simulink model "UAV"  (R2024a)
settings: Solver=FixedStepAuto  StartTime=0  StopTime=inf  MaxStep=0.01  RelTol=1e-4
values from neighbouring files (symbols this model uses):
  actuatorCentres = 0.0    [data.sldd]
  datcom1 : value not decoded    [data.sldd]
  deflectionLimits = -10.0    [data.sldd]
  loggingSampleTime = 1.0    [data.sldd]
  sensorSampleTime = 0.02    [data.sldd]
  vehicle = 1.23    [data.sldd]
undefined symbols (not defined in the file or in its folder): aeroCoeff, aMode, DiscIntNeverNeededParam, Discrete, Earth, HDBK, MIL, Newton, pa28, Raphson, Time, WGS84
libraries: slpidlib x20, simulink_extras x15, simulink x13, arduinolib x8, aerolibasang x5, aerolibactuator x4, aerolibutil x4, aerolibtransform2 x4, sharedtransform x3, ctrlSharedLib x3, aerolibadyn x3, dspstat3 x2
(part 1 of 5)
settings Model: DataDictionary=data.sldd  EnableAccessToBaseWorkspace=off  VariantConfigurationObject=Variants  SnapshotBufferSize=2  SnapshotInterval=1  PacingRate=10  ExtModeTrigDuration=2  Creator=Aliak  LastModifiedBy=abdul
settings SolverCC: AlgebraicLoopSolver=TrustRegion  SolverResetMethod=Robust  MinimalZcImpactIntegration=on
settings OptimizationCC: DefaultParameterBehavior=Inlined  UseDivisionForNetSlopeComputation=on  GainParamInheritBuiltInType=on  UseFloatMulNetSlope=on  DefaultUnderspecifiedDataType=single  UseSpecifiedMinMax=on  InlineInvariantSignals=on  EnhancedBackFolding=on  CachingGlobalReferences=on  ActiveStateOutputEnumStorageType=Smallest  ZeroExternalMemoryAtStartup=off  ZeroInternalMemoryAtStartup=off  EfficientFloat2IntCast=on  EfficientMapNaN2IntZero=off  LifeSpan=0.2  MaxStackSize=64  SimCompilerOptimization=on  OptimizeBlockOrder=speed  DifferentSizesBufferReuse=on  EfficientTunableParamExpr=on
settings DebuggingCC: ConsistencyChecking=warning  ReadBeforeWriteMsg=DisableAll  WriteAfterWriteMsg=DisableAll  WriteAfterReadMsg=DisableAll  SolverPrmCheckMsg=warning  ParameterTunabilityLossMsg=error  UnconnectedInputMsg=warning  UnconnectedOutputMsg=warning  UnconnectedLineMsg=warning  UniqueDataStoreMsg=error  BusObjectLabelMismatch=error  StateNameClashWarn=warning  ForceCombineOutputUpdateInSim=on  ArithmeticOperatorsInVariantConditions=warning
settings HardwareCC: ProdBitPerInt=16  ProdBitPerPointer=16  ProdBitPerSizeT=16  ProdBitPerPtrDiffT=16  ProdLargestAtomicFloat=None  ProdWordSize=8  ProdLongLongMode=on  ProdHWDeviceType=Atmel->AVR  TargetBitPerPointer=64  TargetBitPerSizeT=64  TargetBitPerPtrDiffT=64  TargetLongLongMode=on  TargetIntDivRoundTo=Zero  TargetEndianess=LittleEndian  TargetWordSize=64  TargetHWDeviceType=MATLAB Host
settings ModelReferenceCC: UpdateModelReferenceTargets=IfOutOfDate  EnableRefExpFcnMdlSchedulingChecks=on  EnableParallelModelReferenceBuilds=on  ModelReferenceMinAlgLoopOccurrences=on
settings SFSimCC: SFSimEcho=off  SimParseCustomCode=off  MATLABDynamicMemAlloc=off  CustomCodeUndefinedFunction=UseInterfaceOnly
settings RTWCC: Description=Embedded Coder  SystemTargetFile=ert.tlc  HardwareBoard=Arduino Uno  TemplateMakefile=ert_default_tmf  GenerateReport=on  Toolchain=Arduino AVR  BuildConfiguration=Faster Runs  IncludeHyperlinkInReport=on  LaunchReport=on  GenerateTraceInfo=on  GenerateTraceReport=on  GenerateTraceReportSl=on  GenerateTraceReportSf=on  GenerateTraceReportEml=on  GPUComputeCapability=3.5
settings CodeAppCC: ForceParamTrailComments=on  IgnoreCustomStorageClasses=off  OperatorAnnotations=on  SimulinkDataObjDesc=on  SFDataObjDesc=on  InsertBlockDesc=on
settings ERTTargetCC: TargetLangStandard=C99 (ISO)  CodeReplacementLibrary=GNU C99 extensions  UtilityFuncGeneration=Shared location  CombineSignalStateStructs=on  SuppressErrorStatus=on  SupportNonFinite=off  SupportContinuousTime=on  SupportVariableSizeSignals=on  InlinedParameterPlacement=NonHierarchical

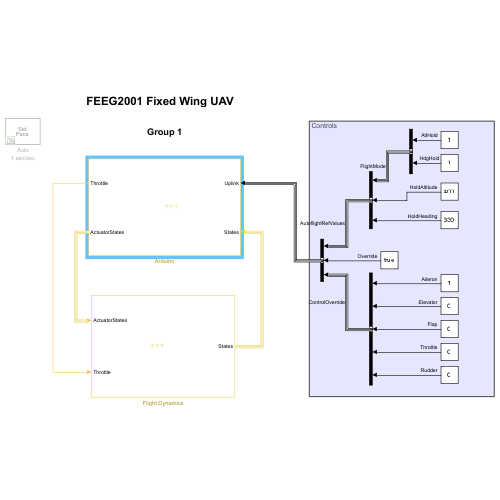
[thumbnail: Simulink's stored preview of the top-level diagram]
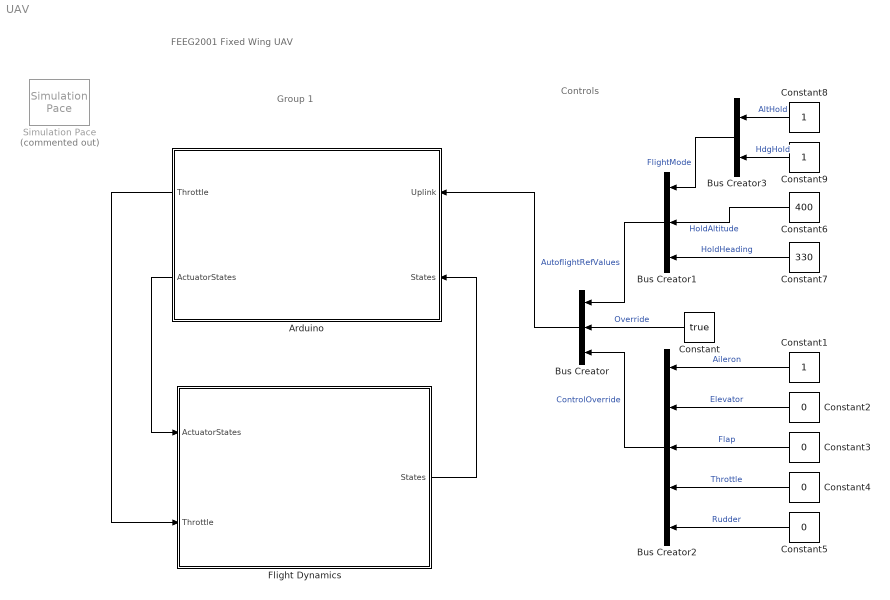
== system UAV ==
  note: Controls
  note: Group 1
  note: FEEG2001 Fixed Wing UAV
  Arduino : Subsystem
      mask Display: image('a000066_featured_1_.jpg');
  Bus Creator : BusCreator  Inputs=3  OutDataTypeStr=Bus: Uplink
  Bus Creator1 : BusCreator  Inputs=3  OutDataTypeStr=Bus: AutoflightDemandedValues
  Bus Creator2 : BusCreator  Inputs=5  OutDataTypeStr=Bus: ControlOverrides
  Bus Creator3 : BusCreator  Inputs=2
  Constant : Constant  Value=true  OutDataTypeStr=boolean
  Constant1 : Constant  OutDataTypeStr=single
  Constant{2..5} (4 alike) : Constant  Value=0  OutDataTypeStr=single
  Constant6 : Constant  Value=400  OutDataTypeStr=single
  Constant7 : Constant  Value=330  OutDataTypeStr=single
  Constant8 : Constant  OutDataTypeStr=single
  Constant9 : Constant  OutDataTypeStr=single
  Flight Dynamics : Subsystem
      mask Display: image('MQ-9-Reaper-armed-UAV.jpg');
  Simulation Pace : aerolibanimutils/Simulation Pace  Commented=on  SimulationPace=1  SleepMode=Auto  OutputPaceError=off  SampleTime=sensorSampleTime
  wires:
  Arduino/2(ActuatorStates) -> Flight Dynamics/1(ActuatorStates)
  Bus Creator/1 -> Arduino/1(Uplink)
  Flight Dynamics/1(States) -> Arduino/2(States)
  Arduino/1(Throttle) -> Flight Dynamics/2(Throttle)
  Bus Creator1/1 -> Bus Creator/1  "AutoflightRefValues"
  Constant/1 -> Bus Creator/2  "Override"
  Bus Creator2/1 -> Bus Creator/3  "ControlOverride"
  Constant1/1 -> Bus Creator2/1  "Aileron"
  Constant2/1 -> Bus Creator2/2  "Elevator"
  Constant3/1 -> Bus Creator2/3  "Flap"
  Constant4/1 -> Bus Creator2/4  "Throttle"
  Constant5/1 -> Bus Creator2/5  "Rudder"
  Bus Creator3/1 -> Bus Creator1/1  "FlightMode"
  Constant6/1 -> Bus Creator1/2  "HoldAltitude"
  Constant7/1 -> Bus Creator1/3  "HoldHeading"
  Constant8/1 -> Bus Creator3/1  "AltHold"
  Constant9/1 -> Bus Creator3/2  "HdgHold"

== system UAV/Arduino ==
  Uplink : Inport
  States : Inport  Port=2
  Actuators : Subsystem  Variant=on  VariantControlMode=label  LabelModeActiveChoice=SimType == 0
  Bus Selector : BusSelector  OutputSignals=Throttle
  Communications : Subsystem
  Flight Control : Subsystem  Variant=on  VariantControlMode=label  VariantControl=Variant1  LabelModeActiveChoice=SimType==0
  Rate Transition : RateTransition  OutPortSampleTime=loggingSampleTime
  Sensors : Subsystem  Variant=on  VariantControlMode=label  VariantControl=Variant1  LabelModeActiveChoice=SimType==0
  Telemetry and Errors : Subsystem  Variant=on  VariantControlMode=label  VariantControl=Variant1  LabelModeActiveChoice=SecArd == 0
  Throttle : Outport  VectorParamsAs1DForOutWhenUnconnected=off
  ActuatorStates : Outport  Port=2  VectorParamsAs1DForOutWhenUnconnected=off
  wires:
  Uplink/1 -> Communications/1(Uplink)
  States/1 -> Sensors/1(States)
  Communications/1(Demands) -> Flight Control/1("Demands ")
  Flight Control/1(" Commands") -> Bus Selector/1, Actuators/1(Commands)
  Rate Transition/1 -> Telemetry and Errors/1("Sensors ")
  Bus Selector/1 -> Throttle/1  "<Throttle>"
  Actuators/1(ActuatorStates) -> ActuatorStates/1
  Sensors/1(" Sensors") -> Flight Control/2("Sensors "), Rate Transition/1

== system UAV/Flight Dynamics ==
  ActuatorStates : Inport
  Throttle : Inport  Port=2
  6DOF EOM : Subsystem  VariantControl=eom3DOF
  Coeff Model : Subsystem  Commented=on  VariantControl=AeroModel==2
  DATCOM Model : Subsystem  TreatAsAtomicUnit=on  VariantControl=AeroModel==1
      settings: MinAlgLoopOccurrences=on
  Environment : Subsystem
  Propulsion : Subsystem
      settings: RTWSystemCode=Inline
  Sum1 : Sum  Inputs=|++  InputSameDT=on  SaturateOnIntegerOverflow=on  OutDataTypeStr=Inherit: Same as first input
  Sum2 : Sum  Inputs=|++  InputSameDT=on  SaturateOnIntegerOverflow=on  OutDataTypeStr=Inherit: Same as first input
  Visualization : Subsystem
  States : Outport  OutDataTypeStr=Bus: States  VectorParamsAs1DForOutWhenUnconnected=off
  wires:
  Sum2/1 -> 6DOF EOM/2(Forces)
  Propulsion/1(F) -> Sum2/2
  Propulsion/2(M) -> Sum1/2
  Sum1/1 -> 6DOF EOM/3(Moments)
  Throttle/1 -> Propulsion/1(cmd)
  ActuatorStates/1 -> DATCOM Model/3(ActuatorStates)
  DATCOM Model/1(F) -> Sum2/1
  DATCOM Model/2(M) -> Sum1/1
  Environment/1(Env) -> 6DOF EOM/1(Env), DATCOM Model/1(Env)
  6DOF EOM/1(DCMbe) -> Environment/2(DCMbe)
  6DOF EOM/2(States) -> Environment/1(States), Visualization/1(States), DATCOM Model/2(States), States/1

== system UAV/Arduino/Actuators ==
  Commands : Inport
  Model Actuators : Subsystem  VariantControl=SimType == 0
  Real Actuators : Subsystem  VariantControl=SimType == 1
  ActuatorStates : Outport  VectorParamsAs1DForOutWhenUnconnected=off

== system UAV/Arduino/Communications ==
  Uplink : Inport  OutDataTypeStr=Bus: Uplink
  Bus Creator : BusCreator  Inputs=5  OutDataTypeStr=Bus: Demands
      settings: InheritFromInputs=off
  Bus Selector : BusSelector  OutputSignals=AutoflightRefValues,Override,ControlOverride
  Bus Selector1 : BusSelector  OutputSignals=FlightMode,HoldAltitude,HoldHeading
  Demands : Outport  OutDataTypeStr=Bus: Demands  VectorParamsAs1DForOutWhenUnconnected=off
  wires:
  Uplink/1 -> Bus Selector/1
  Bus Selector/1 -> Bus Selector1/1  "<AutoflightRefValues>"
  Bus Selector1/1 -> Bus Creator/1  "<FlightMode>"
  Bus Selector1/2 -> Bus Creator/2  "<HoldAltitude>"
  Bus Selector1/3 -> Bus Creator/3  "<HoldHeading>"
  Bus Creator/1 -> Demands/1
  Bus Selector/3 -> Bus Creator/5  "<ControlOverride>"
  Bus Selector/2 -> Bus Creator/4  "<Override>"

== system UAV/Arduino/Flight Control ==
  "Demands " : Inport
  "Sensors " : Inport  Port=2
  Model Flight Control : Subsystem  VariantControl=SimType==0
  Real Flight Control : Subsystem  VariantControl=SimType==1
  " Commands" : Outport  VectorParamsAs1DForOutWhenUnconnected=off

== system UAV/Arduino/Sensors ==
  States : Inport
  Model Sensors : Subsystem  VariantControl=SimType==0
  Real Sensors : Subsystem  VariantControl=SimType==1
  " Sensors" : Outport  OutDataTypeStr=Bus: Sensors  VectorParamsAs1DForOutWhenUnconnected=off

== system UAV/Arduino/Telemetry and Errors ==
  "Sensors " : Inport  OutDataTypeStr=Bus: Sensors  SampleTime=loggingSampleTime
  SD_Logging : Subsystem  VariantControl=SecArd == 1
  Simulink Logging : Subsystem  VariantControl=SecArd == 0

== system UAV/Flight Dynamics/6DOF EOM ==
  Bus Element In : Inport  PortName=Env  Element=g
  Forces : Inport  Port=2
  Moments : Inport  Port=3
  6DOF (Euler Angles) : shared6dof/6DOF (Euler Angles)  units=Metric (MKS)  mtype=Fixed  rep=Quaternion  xme_0=initConditions.x0  Vm_0=initConditions.v0  eul_0=initConditions.euler0  pm_0=initConditions.w0  mass_0=vehicle.mass  mass_e=0.5  mass_f=2.0  inertia=vehicle.inertia  inertia_e=eye(3)  inertia_f=2*eye(3)  k_quat=1.0  vre_flag=on  abi_flag=on  aMode=0  xme_statename=''  Vm_statename=''  eul_statename=''  quat_statename=''  pm_statename=''  mass_statename=''
  Cast To Double : DataTypeConversion  OutDataTypeStr=double  SaturateOnIntegerOverflow=off  RndMeth=Floor
  Gain : Gain  Gain=vehicle.mass
  Product : Product  Multiplication=Matrix(*)
  Sum2 : Sum  Inputs=++|  InputSameDT=on  SaturateOnIntegerOverflow=on  OutDataTypeStr=Inherit: Same as first input
  Terminator1 : Terminator
  DCMbe : Outport  VectorParamsAs1DForOutWhenUnconnected=off
  Bus Element Out : Outport  Port=2  VectorParamsAs1DForOutWhenUnconnected=off  PortName=States  Element=phi_theta_psi
  Bus Element Out1 : Outport  Port=2  VectorParamsAs1DForOutWhenUnconnected=off  PortName=States  Element=pqr
  Bus Element Out2 : Outport  Port=2  VectorParamsAs1DForOutWhenUnconnected=off  PortName=States  Element=omega_dot
  Bus Element Out15 : Outport  Port=2  VectorParamsAs1DForOutWhenUnconnected=off  PortName=States  Element=X_e
  Bus Element Out16 : Outport  Port=2  VectorParamsAs1DForOutWhenUnconnected=off  PortName=States  Element=V_b
  Bus Element Out17 : Outport  Port=2  VectorParamsAs1DForOutWhenUnconnected=off  PortName=States  Element=A_be
  Bus Element Out3 : Outport  Port=2  VectorParamsAs1DForOutWhenUnconnected=off  PortName=States  Element=V_e
  wires:
  6DOF (Euler Angles)/4 -> DCMbe/1, Product/1
  6DOF (Euler Angles)/1 -> Cast To Double/1
  Bus Element In/1 -> Gain/1
  6DOF (Euler Angles)/9 -> Bus Element Out17/1
  6DOF (Euler Angles)/7 -> Bus Element Out2/1
  6DOF (Euler Angles)/6 -> Bus Element Out1/1
  6DOF (Euler Angles)/5 -> Bus Element Out16/1
  6DOF (Euler Angles)/3 -> Bus Element Out/1
  6DOF (Euler Angles)/2 -> Bus Element Out15/1
  Gain/1 -> Product/2
  Sum2/1 -> 6DOF (Euler Angles)/1
  Product/1 -> Sum2/1
  6DOF (Euler Angles)/8 -> Terminator1/1
  Moments/1 -> 6DOF (Euler Angles)/2
  Forces/1 -> Sum2/2
  Cast To Double/1 -> Bus Element Out3/1

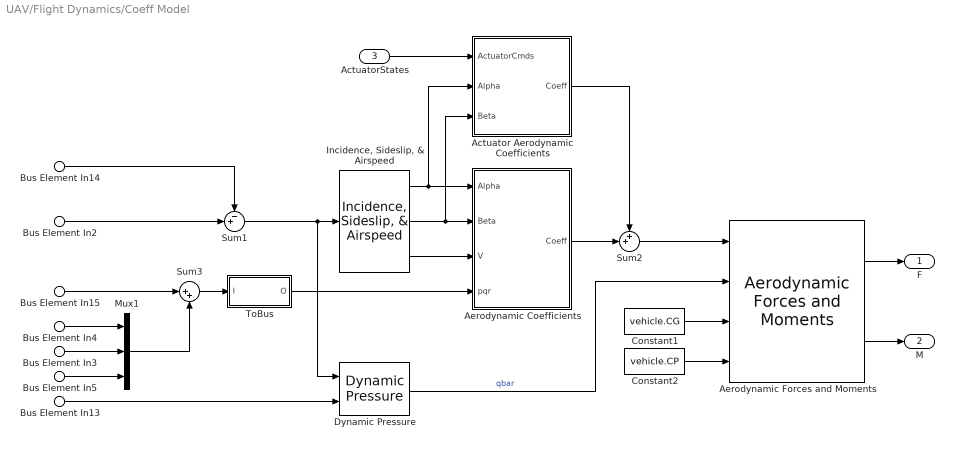
== system UAV/Flight Dynamics/Coeff Model ==
  Bus Element In13 : Inport  PortName=Env  Element=AirDensity
  Bus Element In14 : Inport  PortName=Env  Element=WindVelocity
  Bus Element In15 : Inport  PortName=Env  Element=WindAngularRates
  Bus Element In3 : Inport  Port=2  PortName=States  Element=q
  Bus Element In4 : Inport  Port=2  PortName=States  Element=p
  Bus Element In5 : Inport  Port=2  PortName=States  Element=r
  Bus Element In2 : Inport  Port=2  PortName=States  Element=V_e
  ActuatorStates : Inport  Port=3  OutDataTypeStr=Bus: ActuatorStates
  Actuator Aerodynamic Coefficients : Subsystem
  Aerodynamic Coefficients : Subsystem
  Aerodynamic Forces and Moments : aerolibadyn/Aerodynamic Forces and Moments   inputAxes=Body  outputForceAxes=Body  outputMomentAxes=Body  S=vehicle.wingarea  b=vehicle.wingspan  cbar=vehicle.aclength
  Constant1 : Constant  Value=vehicle.CG
  Constant2 : Constant  Value=vehicle.CP
  Dynamic Pressure : aerolibasang/Dynamic Pressure
  "Incidence, Sideslip, & Airspeed" : aerolibasang/Incidence, Sideslip, & Airspeed
  Mux1 : Mux  Inputs=3
  Sum1 : Sum  Inputs=-+|  InputSameDT=on  SaturateOnIntegerOverflow=on  OutDataTypeStr=Inherit: Same as first input
  Sum2 : Sum  Inputs=++|
  Sum3 : Sum  Inputs=|++  InputSameDT=on  SaturateOnIntegerOverflow=on  OutDataTypeStr=Inherit: Same as first input
  ToBus : Subsystem
  F : Outport  Unit=N  VectorParamsAs1DForOutWhenUnconnected=off
  M : Outport  Port=2  Unit=N*m  VectorParamsAs1DForOutWhenUnconnected=off
  wires:
  ActuatorStates/1 -> Actuator Aerodynamic Coefficients/1(ActuatorCmds)
  Bus Element In14/1 -> Sum1/1
  Bus Element In2/1 -> Sum1/2
  Mux1/1 -> Sum3/2
  Bus Element In15/1 -> Sum3/1
  Bus Element In5/1 -> Mux1/3
  Bus Element In3/1 -> Mux1/2
  Bus Element In4/1 -> Mux1/1
  Actuator Aerodynamic Coefficients/1(Coeff) -> Sum2/1
  Aerodynamic Coefficients/1(Coeff) -> Sum2/2
  ToBus/1(O) -> Aerodynamic Coefficients/4(pqr)
  Sum1/1 -> Dynamic Pressure/1, "Incidence, Sideslip, & Airspeed"/1
  Dynamic Pressure/1 -> Aerodynamic Forces and Moments/2  "qbar"
  Sum3/1 -> ToBus/1(I)
  Bus Element In13/1 -> Dynamic Pressure/2
  "Incidence, Sideslip, & Airspeed"/3 -> Aerodynamic Coefficients/3(V)
  "Incidence, Sideslip, & Airspeed"/2 -> Aerodynamic Coefficients/2(Beta), Actuator Aerodynamic Coefficients/3(Beta)
  Aerodynamic Forces and Moments/2 -> M/1
  Aerodynamic Forces and Moments/1 -> F/1
  Constant2/1 -> Aerodynamic Forces and Moments/4
  Constant1/1 -> Aerodynamic Forces and Moments/3
  Sum2/1 -> Aerodynamic Forces and Moments/1
  "Incidence, Sideslip, & Airspeed"/1 -> Actuator Aerodynamic Coefficients/2(Alpha), Aerodynamic Coefficients/1(Alpha)

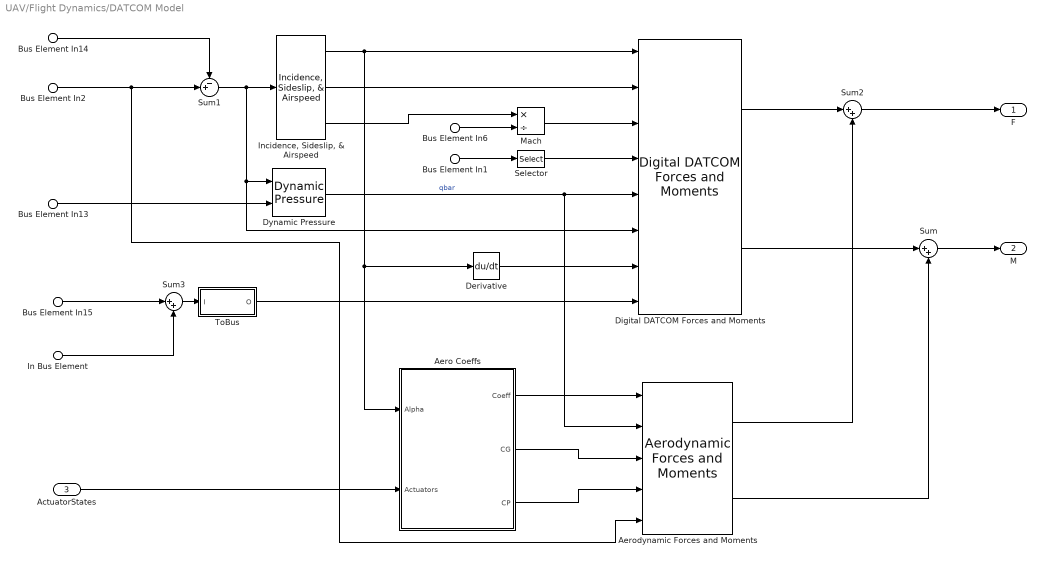
== system UAV/Flight Dynamics/DATCOM Model ==
  Bus Element In13 : Inport  PortName=Env  Element=AirDensity
  Bus Element In14 : Inport  PortName=Env  Element=WindVelocity
  Bus Element In15 : Inport  PortName=Env  Element=WindAngularRates
  Bus Element In6 : Inport  PortName=Env  Element=a
  Bus Element In2 : Inport  Port=2  PortName=States  Element=V_e
  Bus Element In1 : Inport  Port=2  PortName=States  Element=X_e
  In Bus Element : Inport  Port=2  PortName=States  Element=pqr
  ActuatorStates : Inport  Port=3  OutDataTypeStr=Bus: ActuatorStates
  Aero Coeffs : Subsystem
  "Aerodynamic Forces and Moments " : aerolibadyn/Aerodynamic Forces and Moments   inputAxes=Wind  outputForceAxes=Body  outputMomentAxes=Body  S=vehicle.wingarea  b=vehicle.wingspan  cbar=vehicle.cbar
  Derivative : Derivative  CoefficientInTFapproximation=1
  Digital DATCOM Forces and Moments : aerolibadyn/Digital DATCOM Forces and Moments  units=Metric (MKS)  dcase=datcom1{3}  fmode=Body  buildno=0  imethod=Linear  emethod=Linear  rmethod=Linear Extrapolation  action=Warning
  Dynamic Pressure : aerolibasang/Dynamic Pressure
  "Incidence, Sideslip, & Airspeed" : aerolibasang/Incidence, Sideslip, & Airspeed
  Mach : Product  Inputs=*/
  Selector : Selector  IndexMode=Zero-based  InputPortWidth=3  IndexOptions=Index vector (dialog)  Indices=[2]  OutputSizes=1
  Sum : Sum  Inputs=|++
  Sum1 : Sum  Inputs=-+|  InputSameDT=on  SaturateOnIntegerOverflow=on  OutDataTypeStr=Inherit: Same as first input
  Sum2 : Sum  Inputs=|++
  Sum3 : Sum  Inputs=|++  InputSameDT=on  SaturateOnIntegerOverflow=on  OutDataTypeStr=Inherit: Same as first input
  ToBus : Subsystem
  F : Outport  Unit=N  VectorParamsAs1DForOutWhenUnconnected=off
  M : Outport  Port=2  Unit=N*m  VectorParamsAs1DForOutWhenUnconnected=off
  wires:
  Bus Element In14/1 -> Sum1/1
  Bus Element In2/1 -> "Aerodynamic Forces and Moments "/5, Sum1/2
  In Bus Element/1 -> Sum3/2
  Bus Element In15/1 -> Sum3/1
  Sum1/1 -> "Incidence, Sideslip, & Airspeed"/1, Digital DATCOM Forces and Moments/6, Dynamic Pressure/1
  Sum3/1 -> ToBus/1(I)
  Bus Element In13/1 -> Dynamic Pressure/2
  "Incidence, Sideslip, & Airspeed"/3 -> Mach/1
  Digital DATCOM Forces and Moments/2 -> Sum/1
  Digital DATCOM Forces and Moments/1 -> Sum2/1
  Dynamic Pressure/1 -> "Aerodynamic Forces and Moments "/2, Digital DATCOM Forces and Moments/5  "qbar"
  Bus Element In1/1 -> Selector/1
  Selector/1 -> Digital DATCOM Forces and Moments/4
  Bus Element In6/1 -> Mach/2
  ActuatorStates/1 -> Aero Coeffs/2(Actuators)
  "Incidence, Sideslip, & Airspeed"/2 -> Digital DATCOM Forces and Moments/2
  "Incidence, Sideslip, & Airspeed"/1 -> Digital DATCOM Forces and Moments/1, Derivative/1, Aero Coeffs/1(Alpha)
  Aero Coeffs/1(Coeff) -> "Aerodynamic Forces and Moments "/1
  Aero Coeffs/2(CG) -> "Aerodynamic Forces and Moments "/3
  Aero Coeffs/3(CP) -> "Aerodynamic Forces and Moments "/4
  Sum/1 -> M/1
  "Aerodynamic Forces and Moments "/2 -> Sum/2
  Sum2/1 -> F/1
  "Aerodynamic Forces and Moments "/1 -> Sum2/2
  ToBus/1(O) -> Digital DATCOM Forces and Moments/8
  Derivative/1 -> Digital DATCOM Forces and Moments/7
  Mach/1 -> Digital DATCOM Forces and Moments/3

== system UAV/Flight Dynamics/Environment ==
  States : Inport
  DCMbe : Inport  Port=2
  Bus Creator : BusCreator  Inputs=5
  Bus Selector : BusSelector  OutputSignals=X_e,V_e
  Dryden Wind Turbulence Model (Discrete (-q +r)) : aerolibwind2/Dryden Wind Turbulence Model  (Continuous (+q -r))  units=Metric (MKS)  spec=MIL-HDBK-1797  model=Discrete Dryden (-q +r)  W20=1  Wdeg=250  TurbProb=10^-1  L_high=533.4  Wingspan=1.8  ts=sensorSampleTime  Seed=[23341 23342 23343 23344]  T_on=off
  Lapse Rate Model : aerolibatmos2/ISA Atmosphere Model  useExtended=off  action=Warning  custom=off  viscosityOut=off  g=9.80665  gamma=1.4  R=287.0531  L=0.0065  h_trop=11000  h_strat=20000  rho0=1.225  P0=101325  T0=288.15  h0=0  S=110.4  Tref=273.15  muref=1.716e-5
  Selector : Selector  IndexMode=Zero-based  InputPortWidth=3  IndexOptions=Index vector (dialog)  Indices=[0]  OutputSizes=1
  Selector1 : Selector  IndexMode=Zero-based  InputPortWidth=3  IndexOptions=Index vector (dialog)  Indices=[0]  OutputSizes=1
  Terminator : Terminator
  Terminator1 : Terminator
  g : Constant  Value=[0 0 9.80665]
  Env : Outport  VectorParamsAs1DForOutWhenUnconnected=off
  wires:
  States/1 -> Bus Selector/1
  Bus Creator/1 -> Env/1
  Selector/1 -> Dryden Wind Turbulence Model (Discrete (-q +r))/1, Lapse Rate Model/1
  Bus Selector/1 -> Selector/1  "<X_e>"
  Lapse Rate Model/4 -> Bus Creator/2  "AirDensity"
  Lapse Rate Model/2 -> Bus Creator/1  "a"
  g/1 -> Bus Creator/3  "g"
  DCMbe/1 -> Dryden Wind Turbulence Model (Discrete (-q +r))/3
  Bus Selector/2 -> Selector1/1  "<V_e>"
  Selector1/1 -> Dryden Wind Turbulence Model (Discrete (-q +r))/2
  Dryden Wind Turbulence Model (Discrete (-q +r))/1 -> Bus Creator/4  "WindVelocity"
  Dryden Wind Turbulence Model (Discrete (-q +r))/2 -> Bus Creator/5  "WindAngularRates"
  Lapse Rate Model/1 -> Terminator/1
  Lapse Rate Model/3 -> Terminator1/1

== system UAV/Flight Dynamics/Propulsion ==
  cmd : Inport  OutDataTypeStr=single
  Cast To Double : DataTypeConversion  OutDataTypeStr=double  SaturateOnIntegerOverflow=off  RndMeth=Floor
  Mux : Mux  Inputs=[1 2]
  Product : Product
  ThrustX : Lookup_n-D  NumberOfTableDimensions=1  LookupTableObject=''  BreakpointsForDimension1=(1/6)*(3+([-3:3]))  IndexSearchMethod=Linear search  BeginIndexSearchUsingPreviousIndexResult=on  Table=vehicle.thrust*(1+tanh([-3:3]))  ExtrapMethod=Clip  InternalRulePriority=Speed  InputSameDT=off
  ThrustYZ : Constant  Value=[0 0]'  SampleTime=-1
  Thrust_M1 : Constant  Value=[0 -0.06 0]  VectorParams1D=off  SampleTime=-1
  Vector Concatenate : Concatenate
  F : Outport  Unit=N  VectorParamsAs1DForOutWhenUnconnected=off
  M : Outport  Port=2  Unit=N*m  VectorParamsAs1DForOutWhenUnconnected=off
  wires:
  Thrust_M1/1 -> Product/2
  ThrustX/1 -> Mux/1, Vector Concatenate/2
  ThrustYZ/1 -> Vector Concatenate/1, Mux/2
  Mux/1 -> F/1
  cmd/1 -> Cast To Double/1
  Product/1 -> M/1
  Vector Concatenate/1 -> Product/1
  Cast To Double/1 -> ThrustX/1

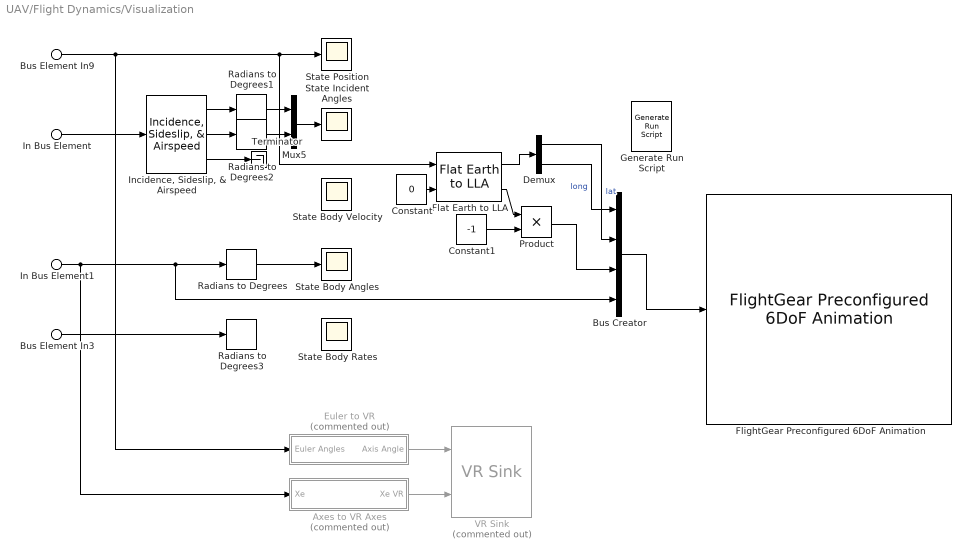
== system UAV/Flight Dynamics/Visualization ==
  Bus Element In3 : Inport  PortName=States  Element=pqr
  In Bus Element : Inport  PortName=States  Element=V_e
  In Bus Element1 : Inport  PortName=States  Element=phi_theta_psi
  Bus Element In9 : Inport  PortName=States  Element=X_e
  Axes to VR Axes : Subsystem  Commented=on
  Bus Creator : BusCreator  Inputs=4
  Constant : Constant  Value=0
  Constant1 : Constant  Value=-1
  Demux : Demux  Outputs=2
  Euler to VR : Subsystem  Commented=on
  Flat Earth to LLA : aerolibtransform2/Flat Earth to LLA  units=Metric (MKS)  ptype=Earth (WGS84)  F=1/298.257223563  R=6378137  refPosPort=off  LL0=[32.2476 15.1232]  psi=0
  FlightGear Preconfigured 6DoF Animation : aerolibfltsims/FlightGear Preconfigured 6DoF Animation  xFlightGearVersion=v2019.1  DestinationIpAddress=127.0.0.1  DestinationPort=5502  SampleTime=1/30  packetVersion=24
  Generate Run Script : aerolibfltsims/Generate Run Script  Architecture=Default  dataFlow=Send  GeometryModelName=pa28-161  AirportId=HL76  RunwayId=33  InitialAltitude=40  InitialHeading=330  OffsetDistance=0  OffsetAzimuth=0  InstallScenery=off  DisableShaders=off  OriginAddress=127.0.0.1  DestinationPort=5502  OriginPort=5505  LocalAddress=127.0.0.1  OutputFileName=runfg.bat  FlightGearBaseDirectory=E:\FlightGear 2020.3
  "Incidence, Sideslip, & Airspeed" : aerolibasang/Incidence, Sideslip, & Airspeed
  Mux5 : Mux  Inputs=2
  Product : Product
  Radians to Degrees{,1..3} (4 alike) : simulink_extras/Transformations/Radians to Degrees
  State Body Angles : Scope
  State Body Rates : Scope
  State Body Velocity : Scope
  State Incident Angles : Scope
  State Position : Scope
  Terminator : Terminator
  VR Sink : vrlib/VR Sink  Commented=on  InstantiateOnLoad=on  SampleTime=0.1  ViewEnable=on  RemoteChange=off  RemoteView=off  FieldsWritten=HL20.rotation.4.1.1.double#HL20.translation.3.1.1.double  WorldFileName=aeroblk_HL20.wrl  WorldDescription=aeroblk_HL20  AutoView=on  VideoDimensions=[]  AllowVariableSize=off  FigureProperties=[]
  wires:
  Mux5/1 -> State Incident Angles/1
  "Incidence, Sideslip, & Airspeed"/2 -> Radians to Degrees2/1
  "Incidence, Sideslip, & Airspeed"/1 -> Radians to Degrees1/1
  In Bus Element/1 -> "Incidence, Sideslip, & Airspeed"/1
  Bus Element In3/1 -> Radians to Degrees3/1
  "Incidence, Sideslip, & Airspeed"/3 -> Terminator/1
  Axes to VR Axes/1(Xe VR) -> VR Sink/2
  In Bus Element1/1 -> Bus Creator/4, Radians to Degrees/1, Axes to VR Axes/1(Xe)
  Euler to VR/1(Axis Angle) -> VR Sink/1
  Bus Element In9/1 -> Flat Earth to LLA/1, State Position/1, Euler to VR/1(Euler Angles)
  Radians to Degrees/1 -> State Body Angles/1
  Radians to Degrees1/1 -> Mux5/1
  Radians to Degrees2/1 -> Mux5/2
  Bus Creator/1 -> FlightGear Preconfigured 6DoF Animation/1
  Constant/1 -> Flat Earth to LLA/2
  Flat Earth to LLA/1 -> Demux/1
  Demux/1 -> Bus Creator/2  "lat"
  Demux/2 -> Bus Creator/1  "long"
  Constant1/1 -> Product/2
  Flat Earth to LLA/2 -> Product/1
  Product/1 -> Bus Creator/3

== system UAV/Arduino/Actuators/Model Actuators ==
  Commands : Inport
  Bus Creator : BusCreator  Inputs=4  OutDataTypeStr=Bus: ActuatorStates
  Bus Selector : BusSelector  OutputSignals=Aileron,Elevator,Rudder,Flap
  Cast To Double{,1..3} (4 alike) : DataTypeConversion  OutDataTypeStr=double  SaturateOnIntegerOverflow=off  RndMeth=Floor
  Constant : Constant  Value=0
  Linear Second-Order Actuator{,1..3} (4 alike) : aerolibactuator/Linear Second-Order Actuator  wn_fin=1  z_fin=0.05  fin_act_0=0  fin_act_vel=0
  Saturation : Saturate  UpperLimit=deflectionLimits.aileron.max  LowerLimit=deflectionLimits.aileron.min
  Saturation1 : Saturate  UpperLimit=deflectionLimits.elevator.max  LowerLimit=deflectionLimits.elevator.min
  Saturation2 : Saturate  UpperLimit=deflectionLimits.rudder.max  LowerLimit=deflectionLimits.rudder.min
  Saturation3 : Saturate  UpperLimit=deflectionLimits.flap.max  LowerLimit=deflectionLimits.flap.min
  Subtract{,1..3} (4 alike) : Sum  Inputs=+-
  ActuatorStates : Outport  VectorParamsAs1DForOutWhenUnconnected=off
  wires:
  Bus Selector/3 -> Subtract2/1  "<Rudder>"
  Bus Selector/4 -> Subtract3/1  "<Flap>"
  Bus Selector/1 -> Subtract1/1  "<Aileron>"
  Bus Selector/2 -> Subtract/1  "<Elevator>"
  Saturation1/1 -> Cast To Double1/1  "Elevator"
  Saturation/1 -> Cast To Double/1  "Aileron"
  Saturation2/1 -> Cast To Double2/1  "Rudder"
  Saturation3/1 -> Cast To Double3/1  "Flap"
  Bus Creator/1 -> ActuatorStates/1
  Commands/1 -> Bus Selector/1
  Subtract1/1 -> Saturation/1
  Subtract/1 -> Saturation1/1
  Subtract2/1 -> Saturation2/1
  Subtract3/1 -> Saturation3/1
  Constant/1 -> Subtract1/2, Subtract/2, Subtract2/2, Subtract3/2
  Cast To Double/1 -> Linear Second-Order Actuator/1
  Cast To Double1/1 -> Linear Second-Order Actuator1/1
  Cast To Double2/1 -> Linear Second-Order Actuator2/1
  Cast To Double3/1 -> Linear Second-Order Actuator3/1
  Linear Second-Order Actuator/1 -> Bus Creator/1  "Aileron"
  Linear Second-Order Actuator1/1 -> Bus Creator/2  "Elevator"
  Linear Second-Order Actuator2/1 -> Bus Creator/3  "Rudder"
  Linear Second-Order Actuator3/1 -> Bus Creator/4  "Flap"

== system UAV/Arduino/Actuators/Real Actuators ==
  Commands : Inport
  Aileron Servos : arduinolib/Standard Servo Write  pinNumber=servoPins.aileron.right  ServoIndex=0  blockPlatform=ARDUINO
  Bus Selector : BusSelector  OutputSignals=AileronCmd,ElevatorCmd,RudderCmd,FlapCmd
  Constant : Constant  Value=actuatorCentres.aileron.left
  Constant1 : Constant  Value=actuatorCentres.elevator.left
  Constant2 : Constant  Value=actuatorCentres.rudder
  Constant3 : Constant  Value=actuatorCentres.flap.left
  Elevator Servo : arduinolib/Standard Servo Write  pinNumber=servoPins.elevator.right  ServoIndex=0  blockPlatform=ARDUINO
  Flap Servo : arduinolib/Standard Servo Write  pinNumber=servoPins.flap.right  ServoIndex=0  blockPlatform=ARDUINO
  Initialize Function : Subsystem  TreatAsAtomicUnit=on
  Rudder Servo : arduinolib/Standard Servo Write  pinNumber=servoPins.rudder  ServoIndex=0  blockPlatform=ARDUINO
  Saturation : Saturate  Commented=through  UpperLimit=deflectionLimits.aileron.max  LowerLimit=deflectionLimits.aileron.min
  Saturation1 : Saturate  Commented=through  UpperLimit=deflectionLimits.elevator.max  LowerLimit=deflectionLimits.elevator.min
  Saturation2 : Saturate  Commented=through  UpperLimit=deflectionLimits.rudder.max  LowerLimit=deflectionLimits.rudder.min
  Saturation3 : Saturate  Commented=through  UpperLimit=deflectionLimits.flap.max  LowerLimit=deflectionLimits.flap.min
  Subtract{,1..3} (4 alike) : Sum  Inputs=-+
  wires:
  Saturation/1 -> Subtract/2
  Bus Selector/3 -> Saturation2/1  "<RudderCmd>"
  Commands/1 -> Bus Selector/1
  Bus Selector/4 -> Saturation3/1  "<FlapCmd>"
  Subtract3/1 -> Flap Servo/1
  Bus Selector/1 -> Saturation/1  "<AileronCmd>"
  Constant2/1 -> Subtract2/1
  Subtract2/1 -> Rudder Servo/1
  Saturation3/1 -> Subtract3/2
  Saturation2/1 -> Subtract2/2
  Saturation1/1 -> Subtract1/2
  Bus Selector/2 -> Saturation1/1  "<ElevatorCmd>"
  Subtract/1 -> Aileron Servos/1
  Subtract1/1 -> Elevator Servo/1
  Constant/1 -> Subtract/1
  Constant1/1 -> Subtract1/1
  Constant3/1 -> Subtract3/1

== system UAV/Arduino/Flight Control/Model Flight Control ==
  Demands : Inport  OutDataTypeStr=Bus: Demands
  Sensors : Inport  Port=2  OutDataTypeStr=Bus: Sensors
  Bus Creator : BusCreator  Inputs=5  OutDataTypeStr=Bus: Commands
      settings: InheritFromInputs=off
  Bus Selector : BusSelector  OutputSignals=ControlOverrides
  Bus Selector2 : BusSelector  OutputSignals=Aileron,Elevator,Flap,Throttle,Rudder
  Bus Selector3 : BusSelector  OutputSignals=Override
  Demux : Demux  Outputs=2
  Guidance States : Stateflow chart  Commented=on
  HDG_ALT : Subsystem
  NOT : Logic  Operator=NOT  IconShape=distinctive  AllPortsSameDT=off  OutDataTypeStr=boolean
  Saturation : Saturate  UpperLimit=deflectionLimits.aileron.max  LowerLimit=deflectionLimits.aileron.min
  Saturation1 : Saturate  UpperLimit=deflectionLimits.elevator.max  LowerLimit=deflectionLimits.elevator.min
  Stabilisation : Subsystem
  Sum : Sum
  Sum1 : Sum
  Switch : Switch  Criteria=u2 ~= 0  SaturateOnIntegerOverflow=off  InputSameDT=off
  Switch1 : Switch  Criteria=u2 ~= 0  SaturateOnIntegerOverflow=off  InputSameDT=off
  Terminator : Terminator
  Terminator1 : Terminator
  Commands : Outport  VectorParamsAs1DForOutWhenUnconnected=off
  wires:
  Bus Creator/1 -> Commands/1
  Sum/1 -> Saturation/1
  Sum1/1 -> Saturation1/1
  Saturation/1 -> Switch/1
  Switch1/1 -> Bus Creator/2  "Elevator"
  Demux/1 -> Sum/2
  Sensors/1 -> HDG_ALT/1(Sensors), Stabilisation/1(Sensors)  "Sensors"
  Demands/1 -> HDG_ALT/2(Demands), Bus Selector3/1, Bus Selector/1  "Demands"
  Bus Selector/1 -> Bus Selector2/1  "<ControlOverrides>"
  Demux/2 -> Sum1/2
  Stabilisation/4(Roll Stab) -> Sum/1
  Stabilisation/3(Pitch Stab) -> Sum1/1
  Stabilisation/2(Yaw Stab) -> Terminator/1
  Bus Selector2/4 -> Bus Creator/4  "<Throttle>"
  Bus Selector2/5 -> Bus Creator/5  "<Rudder>"
  Stabilisation/1(Stall Stab) -> Terminator1/1
  Bus Selector2/3 -> Bus Creator/3  "<Flap>"
  Switch/1 -> Bus Creator/1  "Aileron"
  Bus Selector2/1 -> Switch/3  "<Aileron>"
  Bus Selector2/2 -> Switch1/3  "<Elevator>"
  Saturation1/1 -> Switch1/1  "Elevator"
  Bus Selector3/1 -> NOT/1  "<Override>"
  HDG_ALT/1(Commands) -> Demux/1
  NOT/1 -> Switch/2, Switch1/2

== system UAV/Arduino/Flight Control/Real Flight Control ==
  note: These controls are overriden in hardware and untouchable by the flight computer as per spec
  Demands : Inport  OutDataTypeStr=Bus: Demands
  Sensors : Inport  Port=2  OutDataTypeStr=Bus: Sensors
  Bus Creator : BusCreator  Inputs=5  OutDataTypeStr=Bus: Commands
      settings: InheritFromInputs=off
  Constant : Constant  Value=0
  Constant1 : Constant  Value=0
  Constant2 : Constant  Value=0
  Demux : Demux  Outputs=2
  Guidance : Stateflow chart  TreatAsAtomicUnit=on
  Saturation : Saturate  UpperLimit=deflectionLimits.aileron.max  LowerLimit=deflectionLimits.aileron.min
  Saturation1 : Saturate  UpperLimit=deflectionLimits.elevator.max  LowerLimit=deflectionLimits.elevator.min
  Stabilisation : Subsystem
  Sum : Sum
  Sum1 : Sum  Inputs=+++
  Terminator : Terminator
  Commands : Outport  VectorParamsAs1DForOutWhenUnconnected=off
  wires:
  Bus Creator/1 -> Commands/1
  Sum/1 -> Saturation/1
  Sum1/1 -> Saturation1/1
  Guidance/1(Commands) -> Demux/1
  Demux/1 -> Sum/2
  Sensors/1 -> Stabilisation/1(Sensors), Guidance/1(Sensors)  "Sensors"
  Demands/1 -> Guidance/2(Demands)  "Demands"
  Demux/2 -> Sum1/3
  Stabilisation/2(Roll Stab) -> Sum/1
  Stabilisation/3(Pitch Stab) -> Sum1/1
  Stabilisation/1(Yaw Stab) -> Terminator/1
  Stabilisation/4(Stall Stab) -> Sum1/2
  Saturation/1 -> Bus Creator/1  "Aileron"
  Saturation1/1 -> Bus Creator/2  "Elevator"
  Constant/1 -> Bus Creator/3  "Flap"
  Constant1/1 -> Bus Creator/4  "Throttle"
  Constant2/1 -> Bus Creator/5  "Rudder"

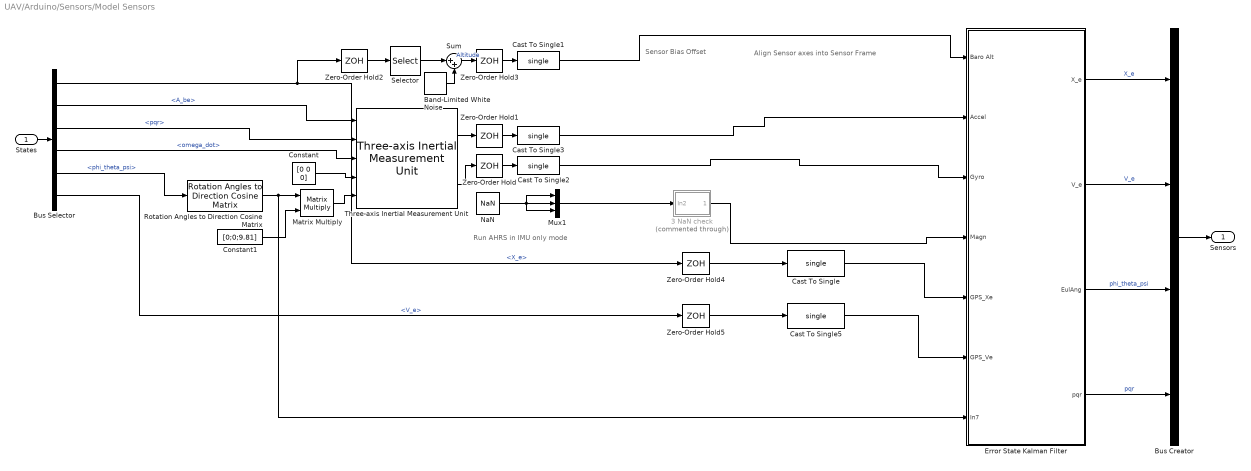
== system UAV/Arduino/Sensors/Model Sensors ==
  note: Run AHRS in IMU only mode
  note: Sensor Bias Offset
  note: Align Sensor axes into Sensor Frame
  States : Inport
  3 NaN check : Subsystem  Commented=through
  Band-Limited White Noise : simulink/Sources/Band-Limited White Noise  Cov=0.001  Ts=sensorSampleTime  seed=[23341]
  Bus Creator : BusCreator  Inputs=4
  Bus Selector : BusSelector  OutputSignals=X_e,A_be,pqr,omega_dot,phi_theta_psi,V_e
  Cast To Single : DataTypeConversion  OutDataTypeStr=single  RndMeth=Simplest  SaturateOnIntegerOverflow=off
  Cast To Single1 : DataTypeConversion  OutDataTypeStr=single  SaturateOnIntegerOverflow=off  RndMeth=Floor
  Cast To Single2 : DataTypeConversion  OutDataTypeStr=single  SaturateOnIntegerOverflow=off  RndMeth=Floor
  Cast To Single3 : DataTypeConversion  OutDataTypeStr=single  SaturateOnIntegerOverflow=off  RndMeth=Floor
  Cast To Single5 : DataTypeConversion  OutDataTypeStr=single  SaturateOnIntegerOverflow=off
  Constant : Constant  Value=[0 0 0]
  Constant1 : Constant  Value=[0;0;9.81]
  Error State Kalman Filter : Subsystem
  Matrix Multiply : Product  Multiplication=Matrix(*)
  Mux1 : Mux  Inputs=3
  NaN : Constant  Value=NaN  OutDataTypeStr=Inherit: Inherit via back propagation
  Rotation Angles to Direction Cosine Matrix : sharedtransform/Rotation Angles to Direction Cosine Matrix  rotationOrder=ZYX  aMode=aMode
  Selector : Selector  IndexMode=Zero-based  InputPortWidth=3  IndexOptions=Index vector (dialog)  Indices=[2]  OutputSizes=1
  Sum : Sum  Inputs=|++
  Three-axis Inertial Measurement Unit : aerolibnav/Three-axis Inertial Measurement Unit  units=Metric (MKS)  imu=[0 0 0]  i_Ts=sensorSampleTime  dtype_a=off  w_a=190  z_a=0.707  a_sf_cc=[1 0 0; 0 1 0; 0 0 1]  a_bias=[0 0 0]  a_sat="[-inf  -inf  -inf  inf inf inf]"  dtype_g=off  w_g=190  z_g=0.707  g_sf_cc=[1 0 0; 0 1 0; 0 0 1]  g_bias=[0 0 0]  g_sens=[0 0 0]  g_sat="[-inf  -inf  -inf  inf inf inf]"  i_rand=off  i_seeds=[23093 23094 23095 23096 23097 23098]  i_pow=[0.001 0.001 0.001 0.0001 0.0001 0.0001]
  Zero-Order Hold{,1..3} (4 alike) : ZeroOrderHold  SampleTime=sensorSampleTime
  Zero-Order Hold4 : ZeroOrderHold
  Zero-Order Hold5 : ZeroOrderHold
  " Sensors" : Outport  VectorParamsAs1DForOutWhenUnconnected=off
  wires:
  Three-axis Inertial Measurement Unit/2 -> Zero-Order Hold/1
  NaN/1 -> Mux1/1, Mux1/2, Mux1/3
  States/1 -> Bus Selector/1
  Three-axis Inertial Measurement Unit/1 -> Zero-Order Hold1/1
  Bus Selector/2 -> Three-axis Inertial Measurement Unit/1  "<A_be>"
  Bus Selector/3 -> Three-axis Inertial Measurement Unit/2  "<pqr>"
  Bus Selector/4 -> Three-axis Inertial Measurement Unit/3  "<omega_dot>"
  Bus Selector/1 -> Zero-Order Hold2/1, Zero-Order Hold4/1  "<X_e>"
  Band-Limited White Noise/1 -> Sum/2
  Constant/1 -> Three-axis Inertial Measurement Unit/4
  Matrix Multiply/1 -> Three-axis Inertial Measurement Unit/5
  Constant1/1 -> Matrix Multiply/2
  Zero-Order Hold/1 -> Cast To Single2/1
  Zero-Order Hold1/1 -> Cast To Single3/1
  Zero-Order Hold2/1 -> Selector/1
  Selector/1 -> Sum/1
  Rotation Angles to Direction Cosine Matrix/1 -> Error State Kalman Filter/7(In7), Matrix Multiply/1
  Bus Selector/5 -> Rotation Angles to Direction Cosine Matrix/1  "<phi_theta_psi>"
  Cast To Single/1 -> Error State Kalman Filter/5(GPS_Xe)
  Error State Kalman Filter/3(EulAng) -> Bus Creator/3  "phi_theta_psi"
  3 NaN check/1(Out1) -> Error State Kalman Filter/4(Magn)
  Cast To Single3/1 -> Error State Kalman Filter/2(Accel)
  Zero-Order Hold3/1 -> Cast To Single1/1
  Bus Selector/6 -> Zero-Order Hold5/1  "<V_e>"
  Error State Kalman Filter/2(V_e) -> Bus Creator/2  "V_e"
  Cast To Single2/1 -> Error State Kalman Filter/3(Gyro)
  Sum/1 -> Zero-Order Hold3/1  "Altitude"
  Error State Kalman Filter/1(X_e) -> Bus Creator/1  "X_e"
  Mux1/1 -> 3 NaN check/1(In2)
  Error State Kalman Filter/4(pqr) -> Bus Creator/4  "pqr"
  Bus Creator/1 -> " Sensors"/1
  Zero-Order Hold4/1 -> Cast To Single/1
  Zero-Order Hold5/1 -> Cast To Single5/1
  Cast To Single5/1 -> Error State Kalman Filter/6(GPS_Ve)
  Cast To Single1/1 -> Error State Kalman Filter/1(Baro Alt)

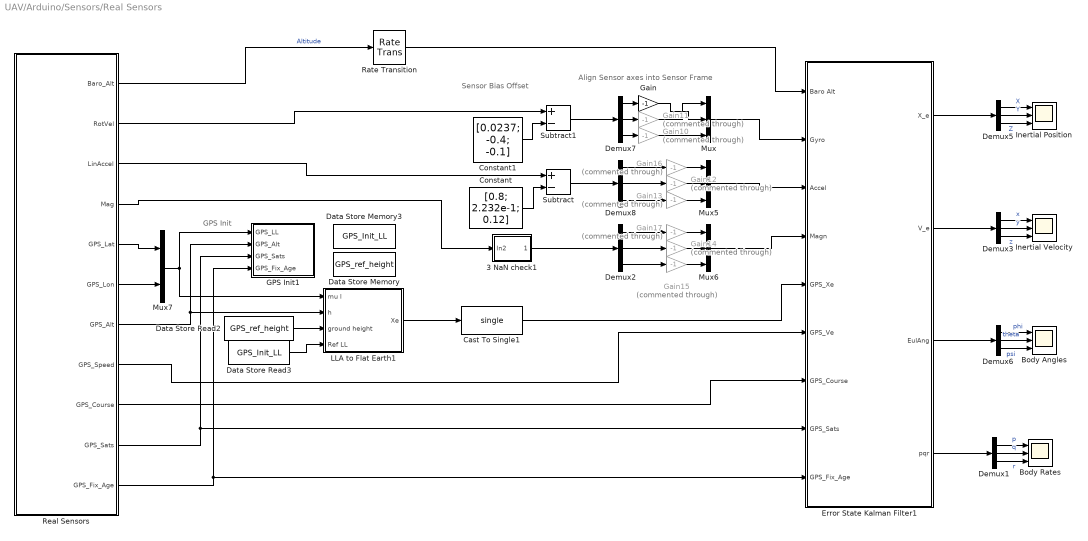
== system UAV/Arduino/Sensors/Real Sensors ==
  note: GPS Init
  note: Align Sensor axes into Sensor Frame
  note: Sensor Bias Offset
  3 NaN check1 : Subsystem
  Body Angles : Scope  NumInputPorts=3
  Body Rates : Scope  NumInputPorts=3
  Cast To Single1 : DataTypeConversion  OutDataTypeStr=single  SaturateOnIntegerOverflow=off  RndMeth=Floor
  Constant : Constant  Value=[0.8; 2.232e-1; 0.12]  VectorParams1D=off
  Constant1 : Constant  Value=[0.0237; -0.4; -0.1]  VectorParams1D=off
  Data Store Memory : DataStoreMemory  DataStoreName=GPS_ref_height  ReadBeforeWriteMsg=warning  WriteAfterWriteMsg=warning  WriteAfterReadMsg=warning  ShowAdditionalParam=off  OutDataTypeStr=single
  Data Store Memory3 : DataStoreMemory  DataStoreName=GPS_Init_LL  ReadBeforeWriteMsg=warning  WriteAfterWriteMsg=warning  WriteAfterReadMsg=warning  InitialValue=[0 0]  ShowAdditionalParam=off  OutDataTypeStr=single
  Data Store Read2 : DataStoreRead  DataStoreName=GPS_ref_height  DataStoreElements=GPS_ref_height  IndexOptions=Index vector (dialog)  Indices=1  OutputSizes=1
  Data Store Read3 : DataStoreRead  DataStoreName=GPS_Init_LL  IndexOptions=Index vector (dialog)  Indices=1  OutputSizes=1
  Demux{1..3,5..8} (7 alike) : Demux  Outputs=3
  Error State Kalman Filter1 : Subsystem
  GPS Init1 : Subsystem
  Gain : Gain  Gain=-1
  Gain{10..13,16} (5 alike) : Gain  Commented=through  Gain=-1
  Gain14 : Gain  Commented=through  Gain=-1  OutDataTypeStr=single
  Gain15 : Gain  Commented=through  Gain=-1  OutDataTypeStr=single
  Gain17 : Gain  Commented=through  Gain=-1  OutDataTypeStr=single
  Inertial Position : Scope  NumInputPorts=3
  Inertial Velocity : Scope  NumInputPorts=3
  LLA to Flat Earth1 : Subsystem
  Mux : Mux  Inputs=3
  Mux5 : Mux  Inputs=3
  Mux6 : Mux  Inputs=3
  Mux7 : Mux  Inputs=2
  Rate Transition : RateTransition
  Real Sensors : Subsystem  VariantControl=SimType==1
  Subtract : Sum  Inputs=+-  OutDataTypeStr=single
  Subtract1 : Sum  Inputs=+-  OutDataTypeStr=single
  wires:
  Real Sensors/1(Baro_Alt) -> Rate Transition/1  "Altitude"
  Real Sensors/5(GPS_Lat) -> Mux7/1
  Real Sensors/3(LinAccel) -> Subtract/1
  Real Sensors/9(GPS_Course) -> Error State Kalman Filter1/7(GPS_Course)
  Real Sensors/10(GPS_Sats) -> GPS Init1/3(GPS_Sats), Error State Kalman Filter1/8(GPS_Sats)
  Real Sensors/11(GPS_Fix_Age) -> GPS Init1/4(GPS_Fix_Age), Error State Kalman Filter1/9(GPS_Fix_Age)
  Gain10/1 -> Mux/3
  Data Store Read3/1 -> LLA to Flat Earth1/4(Ref LL)
  Mux5/1 -> Error State Kalman Filter1/3(Accel)
  Rate Transition/1 -> Error State Kalman Filter1/1(Baro Alt)
  Cast To Single1/1 -> Error State Kalman Filter1/5(GPS_Xe)
  Mux7/1 -> LLA to Flat Earth1/1(mu l), GPS Init1/1(GPS_LL)
  Real Sensors/6(GPS_Lon) -> Mux7/2
  Error State Kalman Filter1/3(EulAng) -> Demux6/1
  Demux6/3 -> Body Angles/3  "psi"
  Real Sensors/4(Mag) -> 3 NaN check1/1(In2)
  Demux3/1 -> Inertial Velocity/1  "x"
  Demux1/3 -> Body Rates/3  "r"
  Error State Kalman Filter1/2(V_e) -> Demux3/1
  Demux6/1 -> Body Angles/1  "phi"
  Demux6/2 -> Body Angles/2  "theta"
  Gain14/1 -> Mux6/2
  Error State Kalman Filter1/1(X_e) -> Demux5/1
  Mux6/1 -> Error State Kalman Filter1/4(Magn)
  Demux8/3 -> Gain13/1
  Gain/1 -> Mux/2
  Data Store Read2/1 -> LLA to Flat Earth1/3(ground height)
  LLA to Flat Earth1/1(Xe) -> Cast To Single1/1
  Demux8/1 -> Gain16/1
  Gain17/1 -> Mux6/1
  Demux2/2 -> Gain14/1
  Demux7/3 -> Gain10/1
  Demux7/2 -> Gain11/1
  3 NaN check1/1(Out1) -> Demux2/1
  Mux/1 -> Error State Kalman Filter1/2(Gyro)
  Demux7/1 -> Gain/1
  Demux8/2 -> Gain12/1
  Demux2/1 -> Gain17/1
  Gain11/1 -> Mux/1
  Gain16/1 -> Mux5/1
  Demux2/3 -> Gain15/1
  Gain15/1 -> Mux6/3
  Gain12/1 -> Mux5/2
  Real Sensors/2(RotVel) -> Subtract1/1
  Real Sensors/7(GPS_Alt) -> LLA to Flat Earth1/2(h), GPS Init1/2(GPS_Alt)
  Demux1/2 -> Body Rates/2  "q"
  Constant1/1 -> Subtract1/2
  Demux3/2 -> Inertial Velocity/2  "y"
  Constant/1 -> Subtract/2
  Subtract1/1 -> Demux7/1
  Demux1/1 -> Body Rates/1  "p"
  Demux3/3 -> Inertial Velocity/3  "z"
  Demux5/3 -> Inertial Position/3  "Z"
  Error State Kalman Filter1/4(pqr) -> Demux1/1
  Real Sensors/8(GPS_Speed) -> Error State Kalman Filter1/6(GPS_Ve)
  Demux5/1 -> Inertial Position/1  "X"
  Gain13/1 -> Mux5/3
  Subtract/1 -> Demux8/1
  Demux5/2 -> Inertial Position/2  "Y"

== system UAV/Arduino/Telemetry and Errors/SD_Logging ==
  "Sensors " : Inport
  Bus Selector : BusSelector  OutputSignals=X_e,V_e,phi_theta_psi,pqr
  Demux{,1..3} (4 alike) : Demux  Outputs=3
  MATLAB System : MATLABSystem  System=SDLogger  SimulateUsing=Code generation
      mask Type: SDLogger
      mask Display:
      | disp('SDLogger');
      | port_label('input',1,'data');
  Vector Concatenate : Concatenate  NumInputs=12
  wires:
  "Sensors "/1 -> Bus Selector/1
  Bus Selector/1 -> Demux/1  "<X_e>"
  Bus Selector/3 -> Demux1/1  "<phi_theta_psi>"
  Bus Selector/4 -> Demux2/1  "<pqr>"
  Bus Selector/2 -> Demux3/1  "<V_e>"
  Vector Concatenate/1 -> MATLAB System/1
  Demux/1 -> Vector Concatenate/1
  Demux/2 -> Vector Concatenate/2
  Demux/3 -> Vector Concatenate/3
  Demux3/1 -> Vector Concatenate/4
  Demux3/2 -> Vector Concatenate/5
  Demux3/3 -> Vector Concatenate/6
  Demux1/1 -> Vector Concatenate/7
  Demux1/2 -> Vector Concatenate/8
  Demux1/3 -> Vector Concatenate/9
  Demux2/1 -> Vector Concatenate/10
  Demux2/2 -> Vector Concatenate/11
  Demux2/3 -> Vector Concatenate/12

== system UAV/Arduino/Telemetry and Errors/Simulink Logging ==
  "Sensors " : Inport  OutDataTypeStr=Bus: Sensors
  Bus Selector : BusSelector  OutputSignals=X_e,V_e,phi_theta_psi,pqr
  Demux{,1..3} (4 alike) : Demux  Outputs=3
  Scope{,1..3} (4 alike) : Scope  NumInputPorts=3
  wires:
  "Sensors "/1 -> Bus Selector/1
  Bus Selector/1 -> Demux/1  "<X_e>"
  Demux/1 -> Scope/1
  Demux/2 -> Scope/2
  Demux/3 -> Scope/3
  Demux1/1 -> Scope1/1
  Demux1/3 -> Scope1/3
  Bus Selector/2 -> Demux1/1  "<V_e>"
  Demux1/2 -> Scope1/2
  Demux2/1 -> Scope2/1
  Demux2/3 -> Scope2/3
  Bus Selector/3 -> Demux2/1  "<phi_theta_psi>"
  Demux2/2 -> Scope2/2
  Demux3/1 -> Scope3/1
  Demux3/3 -> Scope3/3
  Bus Selector/4 -> Demux3/1  "<pqr>"
  Demux3/2 -> Scope3/2

== system UAV/Flight Dynamics/Coeff Model/Actuator Aerodynamic Coefficients ==
  Bus Element In13 : Inport  PortName=ActuatorCmds  Element=Elevator
  Bus Element In1 : Inport  PortName=ActuatorCmds  Element=Aileron
  Bus Element In2 : Inport  PortName=ActuatorCmds  Element=Rudder
  Alpha : Inport  Port=2
  Beta : Inport  Port=3
  Aileron : Subsystem
  Constant : Constant  Value=0
  Elevator : Subsystem
  Flap : Subsystem
  Rudder : Subsystem
  Sum : Sum  Inputs=4  InputSameDT=on  SaturateOnIntegerOverflow=on  OutDataTypeStr=Inherit: Same as first input
  Coeff : Outport  InitialOutput=0  VectorParamsAs1DForOutWhenUnconnected=off
  wires:
  Constant/1 -> Flap/1(Actuator)
  Bus Element In2/1 -> Rudder/1(Actuator)
  Bus Element In1/1 -> Aileron/1(Actuator)
  Bus Element In13/1 -> Elevator/1(Actuator)
  Beta/1 -> Elevator/2(Beta)
  Flap/1(delCoeff) -> Sum/4
  Alpha/1 -> Flap/2(Alpha), Rudder/2(Alpha), Aileron/2(Alpha)
  Rudder/1(delCoeff) -> Sum/3
  Aileron/1(delCoeff) -> Sum/2
  Elevator/1(delCoeff) -> Sum/1
  Sum/1 -> Coeff/1

== system UAV/Flight Dynamics/Coeff Model/Aerodynamic Coefficients ==
  Alpha : Inport
  Beta : Inport  Port=2
  V : Inport  Port=3
  pqr : Inport  Port=4  Unit=m/s
  Body Rate Damping : Subsystem
  Datum Coefficients : Subsystem
  Sum : Sum  Inputs=|++
  Coeff : Outport  VectorParamsAs1DForOutWhenUnconnected=off
  wires:
  pqr/1 -> Body Rate Damping/2(pqr)
  Sum/1 -> Coeff/1
  V/1 -> Body Rate Damping/1(V)
  Body Rate Damping/1(Coeff) -> Sum/2
  Datum Coefficients/1(Coeff) -> Sum/1
  Beta/1 -> Datum Coefficients/2(Beta)
  Alpha/1 -> Datum Coefficients/1(Alpha)

== system UAV/Flight Dynamics/Coeff Model/ToBus ==
  I : Inport
  Bus Creator3 : BusCreator  Inputs=3
  Demux : Demux  Outputs=3
  O : Outport  VectorParamsAs1DForOutWhenUnconnected=off
  wires:
  I/1 -> Demux/1
  Demux/2 -> Bus Creator3/2  "q_wind"
  Bus Creator3/1 -> O/1
  Demux/3 -> Bus Creator3/3  "r_wind"
  Demux/1 -> Bus Creator3/1  "p_wind"

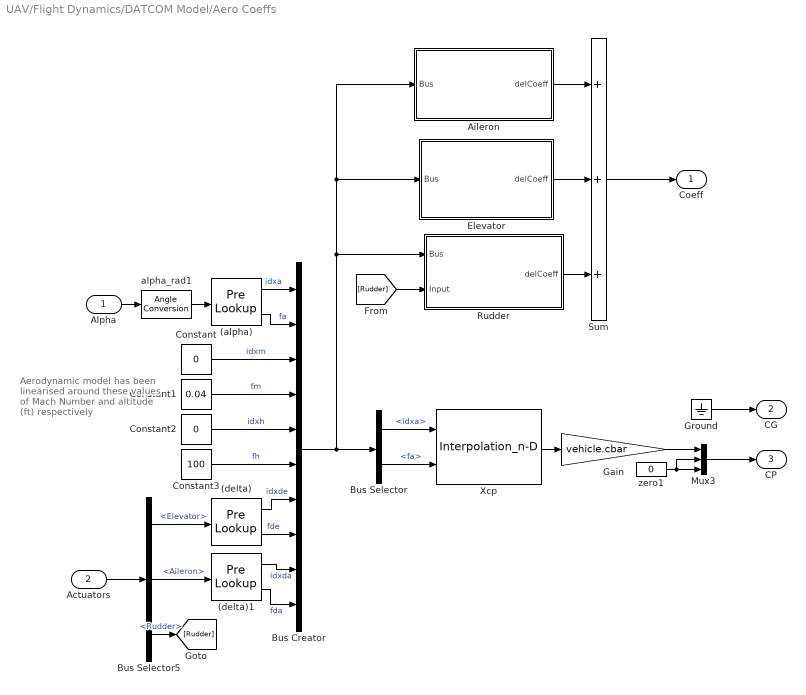
== system UAV/Flight Dynamics/DATCOM Model/Aero Coeffs ==
  note: Aerodynamic model has been linearised around these values of Mach Number and altitude (ft) respectively
  Alpha : Inport
  Actuators : Inport  Port=2
  (alpha) : PreLookup  BreakpointsData=datcom1{3}.alpha  BeginIndexSearchUsingPreviousIndexResult=on  ExtrapMethod=Linear  IndexDataTypeStr=int32  FractionDataTypeStr=double
  (delta) : PreLookup  BreakpointsData=datcom1{3}.delta  BeginIndexSearchUsingPreviousIndexResult=on  ExtrapMethod=Linear  IndexDataTypeStr=int32  FractionDataTypeStr=double
  (delta)1 : PreLookup  BreakpointsData=datcom1{2}.deltal  BeginIndexSearchUsingPreviousIndexResult=on  ExtrapMethod=Linear  IndexDataTypeStr=int32  FractionDataTypeStr=double
  Aileron : Subsystem
  Bus Creator : BusCreator  Inputs=10
  Bus Selector : BusSelector  OutputSignals=idxa,fa
  Bus Selector5 : BusSelector  OutputSignals=Elevator,Aileron,Rudder
  Constant : Constant  Value=0
  Constant1 : Constant  Value=0.04
  Constant2 : Constant  Value=0
  Constant3 : Constant  Value=100
  Elevator : Subsystem
  Gain : Gain  Gain=vehicle.cbar
  Ground : Ground
  Mux3 : Mux  Inputs=3
  Rudder : Subsystem
  Sum : Sum  Inputs=3  InputSameDT=on  SaturateOnIntegerOverflow=on  OutDataTypeStr=Inherit: Same as first input
  Xcp : Interpolation_n-D  NumberOfTableDimensions=1  Table=datcom1{1}.xcp  DiagnosticForOutOfRangeInput=Warning  OutDataTypeStr=double
      settings: InputPortMap=u0,u1
  alpha_rad1 : aerolibconvert2/Angle Conversion  IU=rad  OU=deg
  zero1 : Constant  Value=0
  Coeff : Outport  VectorParamsAs1DForOutWhenUnconnected=off
  CG : Outport  Port=2  PortDimensions=3  VectorParamsAs1DForOutWhenUnconnected=off
  CP : Outport  Port=3  PortDimensions=3  VectorParamsAs1DForOutWhenUnconnected=off
  wires:
  Aileron/1(delCoeff) -> Sum/1
  Sum/1 -> Coeff/1
  (alpha)/1 -> Bus Creator/1  "idxa"
  Gain/1 -> Mux3/1
  (delta)/2 -> Bus Creator/8  "fde"
  (alpha)/2 -> Bus Creator/2  "fa"
  alpha_rad1/1 -> (alpha)/1
  Elevator/1(delCoeff) -> Sum/2
  Alpha/1 -> alpha_rad1/1
  (delta)/1 -> Bus Creator/7  "idxde"
  zero1/1 -> Mux3/2, Mux3/3
  Bus Selector/1 -> Xcp/1  "<idxa>"
  Bus Creator/1 -> Aileron/1(Bus), Elevator/1(Bus), Rudder/1(Bus), Bus Selector/1
  Bus Selector/2 -> Xcp/2  "<fa>"
  Actuators/1 -> Bus Selector5/1
  Constant/1 -> Bus Creator/3  "idxm"
  Constant1/1 -> Bus Creator/4  "fm"
  Rudder/1(delCoeff) -> Sum/3
  Ground/1 -> CG/1
  Mux3/1 -> CP/1
  Xcp/1 -> Gain/1
  Bus Selector5/1 -> (delta)/1  "<Elevator>"
  Bus Selector5/2 -> (delta)1/1  "<Aileron>"
  (delta)1/1 -> Bus Creator/9  "idxda"
  (delta)1/2 -> Bus Creator/10  "fda"
  Constant2/1 -> Bus Creator/5  "idxh"
  Constant3/1 -> Bus Creator/6  "fh"
  [Rudder] -> Rudder/2(Input)
  Bus Selector5/3 -> [Rudder]  "<Rudder>"

== system UAV/Flight Dynamics/DATCOM Model/ToBus ==
  I : Inport
  Bus Creator3 : BusCreator  Inputs=3
  Demux : Demux  Outputs=3
  O : Outport  VectorParamsAs1DForOutWhenUnconnected=off
  wires:
  I/1 -> Demux/1
  Demux/2 -> Bus Creator3/2  "q_wind"
  Bus Creator3/1 -> O/1
  Demux/3 -> Bus Creator3/3  "r_wind"
  Demux/1 -> Bus Creator3/1  "p_wind"

== system UAV/Flight Dynamics/Visualization/Axes to VR Axes ==
  Xe : Inport
  Concatenate : Concatenate  NumInputs=3
  Demux : Demux  Outputs=3
      settings: DisplayOption=none
  rad-->deg : Gain  Gain=-1  SaturateOnIntegerOverflow=on  OutDataTypeStr=Inherit: Same as input  ParamDataTypeStr=Inherit: Same as input
  rad-->deg1 : Gain  Gain=-1  SaturateOnIntegerOverflow=on  OutDataTypeStr=Inherit: Same as input  ParamDataTypeStr=Inherit: Same as input
  Xe VR : Outport  VectorParamsAs1DForOutWhenUnconnected=off
  wires:
  Xe/1 -> Demux/1
  Demux/1 -> Concatenate/1
  Demux/2 -> rad-->deg/1
  Demux/3 -> rad-->deg1/1
  Concatenate/1 -> Xe VR/1
  rad-->deg1/1 -> Concatenate/2
  rad-->deg/1 -> Concatenate/3

== system UAV/Flight Dynamics/Visualization/Euler to VR ==
  Euler Angles : Inport
  Axis Angle Vector : Subsystem
  Demux : Demux  Outputs=3
      settings: DisplayOption=none
  Mux : Mux  Inputs=2
  Mux1 : Mux  Inputs=2
  Mux2 : Mux  Inputs=2
  Quaternion Multiplication (Pitch & Yaw) : aerolibutil/Quaternion Multiplication
  Quaternion Multiplication (Roll) : aerolibutil/Quaternion Multiplication
  Quaternion Normalization : Subsystem
  Quaternion Normalization1 : Subsystem
  Quaternion Normalization2 : Subsystem
  Vr Pitch Axes : Constant  Value=[0 0 1]
  Vr Roll Axes : Constant  Value=[1 0 0]
  Vr Yaw Axes : Constant  Value=[0 -1 0]
  Axis Angle : Outport  VectorParamsAs1DForOutWhenUnconnected=off
  wires:
  Quaternion Multiplication (Roll)/1 -> Axis Angle Vector/1(e0)
  Quaternion Multiplication (Pitch & Yaw)/1 -> Quaternion Multiplication (Roll)/2
  Axis Angle Vector/1(e0_norm) -> Axis Angle/1
  Quaternion Normalization/1(e0_norm) -> Quaternion Multiplication (Roll)/1
  Quaternion Normalization2/1(e0_norm) -> Quaternion Multiplication (Pitch & Yaw)/1
  Quaternion Normalization1/1(e0_norm) -> Quaternion Multiplication (Pitch & Yaw)/2
  Mux2/1 -> Quaternion Normalization2/1(e0)
  Mux1/1 -> Quaternion Normalization1/1(e0)
  Mux/1 -> Quaternion Normalization/1(e0)
  Demux/3 -> Mux2/1
  Vr Yaw Axes/1 -> Mux2/2
  Demux/2 -> Mux1/1
  Vr Pitch Axes/1 -> Mux1/2
  Demux/1 -> Mux/1
  Vr Roll Axes/1 -> Mux/2
  Euler Angles/1 -> Demux/1
